simulink model "Proj_06_11"  (R2020a)
settings: Solver=VariableStepAuto  StartTime=0.0  StopTime=50  MaxStep=1e-3  RelTol=1e-3
undefined symbols (not defined in the file): T
settings Model: Creator=jguil  LastModifiedBy=jguil

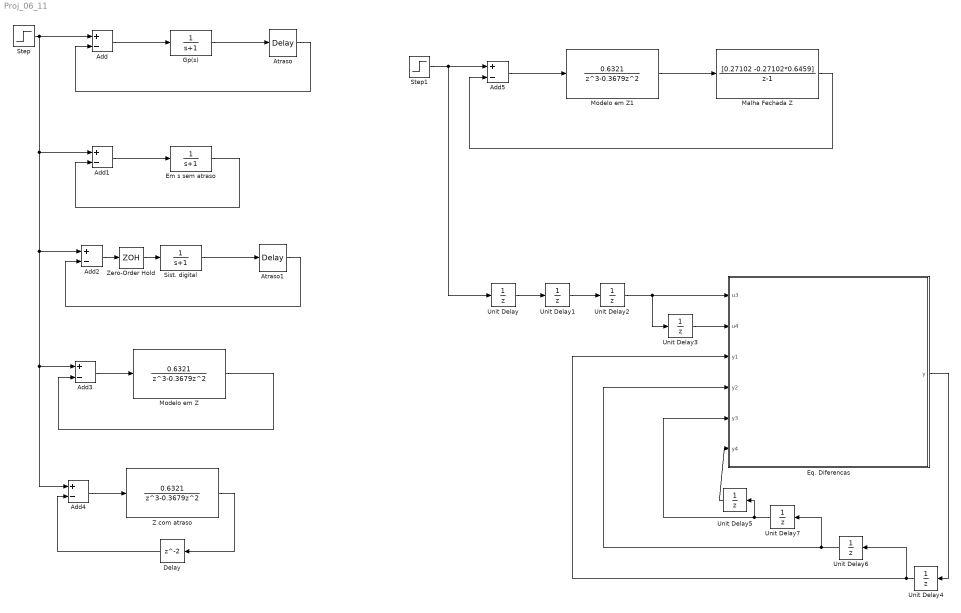
== system Proj_06_11 ==
  Add{,1..5} (6 alike) : Sum  Inputs=+-
  Atraso : TransportDelay  DelayTime=2
  Atraso1 : TransportDelay  DelayTime=2
  Delay : Delay  SampleTime=T
  Em s sem atraso : TransferFcn  Denominator=[1 1]
  Eq. Diferencas : MATLAB Function  TreatAsAtomicUnit=on
  Gp(s) : TransferFcn  Denominator=[1 1]
  Malha Fechada Z : DiscreteTransferFcn  Numerator=[0.27102 -0.27102*0.6459]  Denominator=[1 -1]  SampleTime=T
  Modelo em Z : DiscreteTransferFcn  Numerator=[0.6321]  Denominator=[1 -0.3679 0 0]  SampleTime=T
  Modelo em Z1 : DiscreteTransferFcn  Numerator=[0.6321]  Denominator=[1 -0.3679 0 0]  SampleTime=T
  Sist. digital : TransferFcn  Denominator=[1 1]
  Step : Step  SampleTime=0
  Step1 : Step  SampleTime=0
  Unit Delay{,1..7} (8 alike) : UnitDelay  SampleTime=T  HasFrameUpgradeWarning=on
  Z com atraso : DiscreteTransferFcn  Numerator=[0.6321]  Denominator=[1 -0.3679 0 0]  SampleTime=T
  Zero-Order Hold : ZeroOrderHold  SampleTime=T
  wires:
  Add/1 -> Gp(s)/1
  Gp(s)/1 -> Atraso/1
  Atraso/1 -> Add/2
  Add1/1 -> Em s sem atraso/1
  Em s sem atraso/1 -> Add1/2
  Atraso1/1 -> Add2/2
  Step/1 -> Add4/1, Add3/1, Add2/1, Add1/1, Add/1
  Sist. digital/1 -> Atraso1/1
  Add2/1 -> Zero-Order Hold/1
  Zero-Order Hold/1 -> Sist. digital/1
  Add3/1 -> Modelo em Z/1
  Modelo em Z/1 -> Add3/2
  Z com atraso/1 -> Delay/1
  Add4/1 -> Z com atraso/1
  Delay/1 -> Add4/2
  Step1/1 -> Unit Delay/1, Add5/1
  Add5/1 -> Modelo em Z1/1
  Modelo em Z1/1 -> Malha Fechada Z/1
  Malha Fechada Z/1 -> Add5/2
  Eq. Diferencas/1(y) -> Unit Delay4/1
  Unit Delay4/1 -> Unit Delay6/1, Eq. Diferencas/3(y1)
  Unit Delay6/1 -> Unit Delay7/1, Eq. Diferencas/4(y2)
  Unit Delay7/1 -> Unit Delay5/1, Eq. Diferencas/5(y3)
  Unit Delay5/1 -> Eq. Diferencas/6(y4)
  Unit Delay2/1 -> Eq. Diferencas/1(u3), Unit Delay3/1
  Unit Delay3/1 -> Eq. Diferencas/2(u4)
  Unit Delay/1 -> Unit Delay1/1
  Unit Delay1/1 -> Unit Delay2/1

== matlab function Proj_06_11/Eq. Diferencas ==
  data: u3 input; y output; u4 input; y1 input; y2 input; y3 input; y4 input
function y = aprox(u3,u4,y1,y2,y3,y4)

y = 1.368*y1-0.3679*y2-0.1713*y3+0.1103*y4+0.1713*u3-0.1103*u4;
